simulink model "IBVStrack"  (Simulink 10.0)
settings: Solver=ode45  StartTime=0.0  StopTime=30.0  RelTol=1e-3  EnableMultiTasking=on
undefined symbols (not defined in the file): c, coords, get, GetHMatrix, p, T0c_x, T0o
libraries: vs x16, simulink3 x4
settings Model: Creator=bhisma  LastModifiedBy=bhisma
settings DataIOCC: LimitDataPoints=on  SignalLoggingSaveFormat=ModelDataLogs  SignalLoggingName=sigsOut
settings OptimizationCC: BooleanDataType=off  LifeSpan=auto
settings DebuggingCC: SaveWithParameterizedLinksMsg=none  SignalResolutionControl=TryResolveAllWithWarning  MultiTaskDSMMsg=warning  MultiTaskCondExecSysMsg=none  SFUnexpectedBacktrackingDiag=error  SFNoUnconditionalDefaultTransitionDiag=error  SFExecutionAtInitializationDiag=warning  ArithmeticOperatorsInVariantConditions=error
settings HardwareCC: TargetUnknown=on
settings SFSimCC: SimUseLocalCustomCode=on  CustomCodeUndefinedFunction=FilterOut
settings RTWCC: RTWUseLocalCustomCode=on
settings CodeAppCC: StateflowObjectComments=off
settings GRTTargetCC: TargetLangStandard=C99 (ISO)

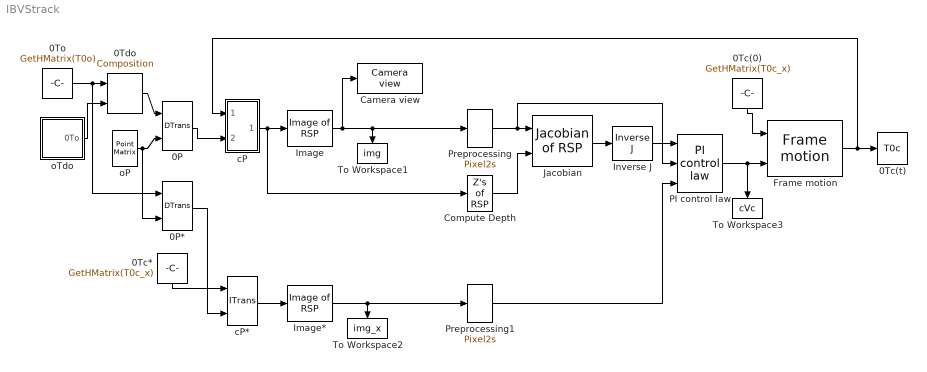
== system IBVStrack ==
  0P : vs/Features/DTrans  SimViewingDevice=off  DataTypeOverride=UseLocalSettings  MinMaxOverflowLogging=UseLocalSettings
      settings: Permissions=ReadWrite  RTWFcnNameOpts=Auto  RTWFileNameOpts=Auto
  0P* : vs/Features/DTrans  SimViewingDevice=off  DataTypeOverride=UseLocalSettings  MinMaxOverflowLogging=UseLocalSettings
      settings: Permissions=ReadWrite  RTWFcnNameOpts=Auto  RTWFileNameOpts=Auto
  0Tc(0) : Constant  Value=GetHMatrix(T0c_x)  VectorParams1D=off
  0Tc(t) : ToWorkspace  VariableName=T0c  SaveFormat=Structure With Time  SampleTime=-1
  0Tc* : Constant  Value=GetHMatrix(T0c_x)  VectorParams1D=off
  0Tdo : vs/Pose/Composition  SimViewingDevice=off  DataTypeOverride=UseLocalSettings  MinMaxOverflowLogging=UseLocalSettings
      settings: Permissions=ReadWrite  RTWFcnNameOpts=Auto  RTWFileNameOpts=Auto
  0To : Constant  Value=GetHMatrix(T0o)  VectorParams1D=off
  Camera view : vs/Camera/Camera view  ms=15  em=normal  umin=0  umax=get(c,'hres')-1  vmin=0  vmax=get(c,'vres')-1  st=-1
  Compute Depth : vs/Features/Z's of RSP  SimViewingDevice=off  DataTypeOverride=UseLocalSettings  MinMaxOverflowLogging=UseLocalSettings
      settings: Permissions=ReadWrite  RTWFcnNameOpts=Auto  RTWFileNameOpts=Auto
  Frame motion : vs/Pose/Frame motion  SimViewingDevice=off  DataTypeOverride=UseLocalSettings  MinMaxOverflowLogging=UseLocalSettings
      settings: Permissions=ReadWrite  RTWFcnNameOpts=Auto  RTWFileNameOpts=Auto
  Image : vs/Camera/Image of RSP  fu=get(c,'fu')  fv=get(c,'fv')  u0=get(c,'u0')  v0=get(c,'v0')
  Image* : vs/Camera/Image of RSP  fu=get(c,'fu')  fv=get(c,'fv')  u0=get(c,'u0')  v0=get(c,'v0')
  Inverse J : vs/Jacobian/Inverse J  SimViewingDevice=off  DataTypeOverride=UseLocalSettings  MinMaxOverflowLogging=UseLocalSettings
      settings: Permissions=ReadWrite  RTWFcnNameOpts=Auto  RTWFileNameOpts=Auto
  Jacobian : vs/Jacobian/Jacobian of RSP  SimViewingDevice=off  DataTypeOverride=UseLocalSettings  MinMaxOverflowLogging=UseLocalSettings
      settings: Permissions=ReadWrite  RTWFcnNameOpts=Auto  RTWFileNameOpts=Auto
  PI control law : vs/Jacobian/PI control law  lambda=5  mu=10
  Preprocessing : vs/Jacobian/Pixel2s  fu=get(c,'fu')  fv=get(c,'fv')  u0=get(c,'u0')  v0=get(c,'v0')
  Preprocessing1 : vs/Jacobian/Pixel2s  fu=get(c,'fu')  fv=get(c,'fv')  u0=get(c,'u0')  v0=get(c,'v0')
  To Workspace1 : ToWorkspace  VariableName=img  SaveFormat=Structure With Time  SampleTime=-1
  To Workspace2 : ToWorkspace  VariableName=img_x  SaveFormat=Structure With Time  SampleTime=-1
  To Workspace3 : ToWorkspace  VariableName=cVc  SaveFormat=Structure With Time  SampleTime=-1
  cP : Subsystem  AncestorBlock=vs/Features/ITrans
  cP* : vs/Features/ITrans  SimViewingDevice=off  DataTypeOverride=UseLocalSettings  MinMaxOverflowLogging=UseLocalSettings
      settings: Permissions=ReadWrite  RTWFcnNameOpts=Auto  RTWFileNameOpts=Auto
  oP : vs/Features/Point Matrix  m=coords(p)
  oTdo : Subsystem
  wires:
  oP/1 -> 0P/2, 0P*/2
  cP/1(bP) -> Compute Depth/1, Image/1
  Image/1 -> Camera view/1, Preprocessing/1, To Workspace1/1
  Preprocessing/1 -> Jacobian/1, PI control law/2
  Compute Depth/1 -> Jacobian/2
  Jacobian/1 -> Inverse J/1
  Inverse J/1 -> PI control law/1
  Preprocessing1/1 -> PI control law/3
  Frame motion/1 -> 0Tc(t)/1, cP/1(aTb)
  0Tc*/1 -> cP*/1
  cP*/1 -> Image*/1
  0P/1 -> cP/2(aP)
  PI control law/1 -> Frame motion/2, To Workspace3/1
  Image*/1 -> Preprocessing1/1, To Workspace2/1
  oTdo/1(0To) -> 0Tdo/2
  0To/1 -> 0P*/1, 0Tdo/1
  0Tdo/1 -> 0P/1
  0P*/1 -> cP*/2
  0Tc(0)/1 -> Frame motion/1

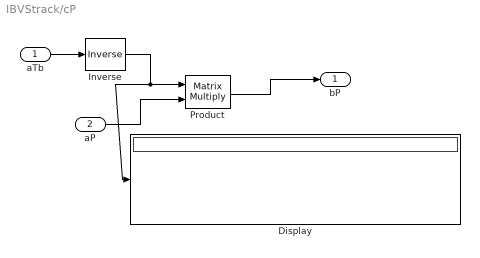
== system IBVStrack/cP ==
  aTb : Inport
  aP : Inport  Port=2
  Display : Display
  Inverse : vs/Pose/Inverse
      settings: RTWFcnNameOpts=Auto  RTWFileNameOpts=Auto
  Product : Product  Multiplication=Matrix(*)  SaturateOnIntegerOverflow=on  InputSameDT=on  OutDataTypeStr=Inherit: Same as first input
  bP : Outport
  wires:
  Inverse/1 -> Product/1, Display/1
  aTb/1 -> Inverse/1
  Product/1 -> bP/1
  aP/1 -> Product/2

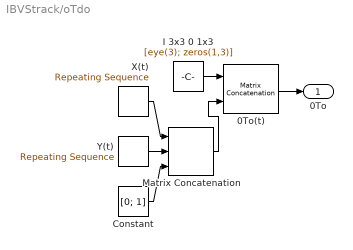
== system IBVStrack/oTdo ==
  0To(t) : simulink3/Signals & Systems/Matrix Concatenation  numInports=2  catMethod=Horizontal
      settings: SourceProductName=Simulink  SourceProductBaseCode=SL
  Constant : Constant  Value=[0; 1]  VectorParams1D=off
  I 3x3 0 1x3 : Constant  Value=[eye(3); zeros(1,3)]  VectorParams1D=off
  Matrix Concatenation : simulink3/Signals & Systems/Matrix Concatenation  numInports=3  catMethod=Vertical
      settings: SourceProductName=Simulink  SourceProductBaseCode=SL
  X(t) : simulink3/Sources/Repeating Sequence  rep_seq_t=[0 1 2 3 4] * 5  rep_seq_y=[0 1 1 0 0] * 0.1
      settings: SourceProductName=Simulink  SourceProductBaseCode=SL
  Y(t) : simulink3/Sources/Repeating Sequence  rep_seq_t=[0 1 2 3 4] * 5  rep_seq_y=[0 0 1 1 0] * 0.1
      settings: SourceProductName=Simulink  SourceProductBaseCode=SL
  0To : Outport
  wires:
  X(t)/1 -> Matrix Concatenation/1
  Matrix Concatenation/1 -> 0To(t)/2
  I 3x3 0 1x3/1 -> 0To(t)/1
  Constant/1 -> Matrix Concatenation/3
  Y(t)/1 -> Matrix Concatenation/2
  0To(t)/1 -> 0To/1
